simulink model "xmc_sobel_edge_detection"  (R2023a)
settings: Solver=VariableStepAuto  StartTime=0.0  StopTime=inf  RelTol=1e-3  EnableMultiTasking=on
PostLoadFcn:
  | xmcHubUpdateInstalledDevice(gcs);
undefined symbols (not defined in the file): A, AXI4, N, Stream, xc7vx485tffg1157
libraries: visionsinks x3, hlsBasic x3, vmcUtilities x2, sobel_edge_detection_lib x2, dspvision x1, hlsUtilities x1
settings Model: Creator=dvancamp  LastModifiedBy=robg
settings SolverCC: AlgebraicLoopSolver=TrustRegion
settings DataIOCC: LimitDataPoints=on  ReturnWorkspaceOutputs=off
settings OptimizationCC: LifeSpan=inf
settings DebuggingCC: UnconnectedInputMsg=warning  UnconnectedOutputMsg=warning  UnconnectedLineMsg=warning  AllowSymbolicDim=off  SFUnexpectedBacktrackingDiag=warning  SFNoUnconditionalDefaultTransitionDiag=warning  ArithmeticOperatorsInVariantConditions=warning
settings ModelReferenceCC: EnableRefExpFcnMdlSchedulingChecks=on  PropagateSignalLabelsOutOfModel=off
settings SFSimCC: SimUseLocalCustomCode=off  CustomCodeUndefinedFunction=UseInterfaceOnly
settings RTWCC: RTWUseLocalCustomCode=off  DLArmComputeVersion=19.05
settings CodeAppCC: StateflowObjectComments=on
settings GRTTargetCC: TargetLangStandard=C89/C90 (ANSI)
settings ConfigComp: CovMetricSettings=dw  CovSaveCumulativeToWorkspaceVar=on  CovSaveSingleToWorkspaceVar=on  CovExternalEMLEnable=off

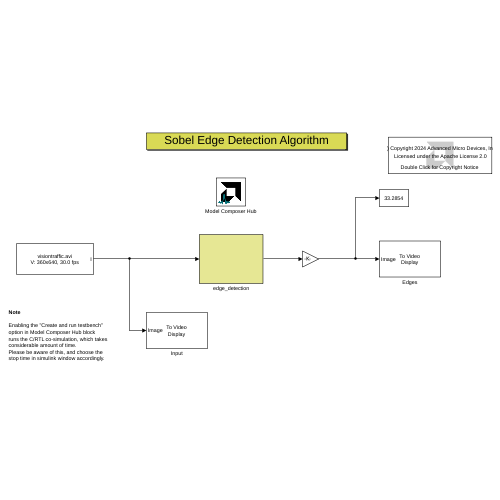
[thumbnail: Simulink's stored preview of the top-level diagram]
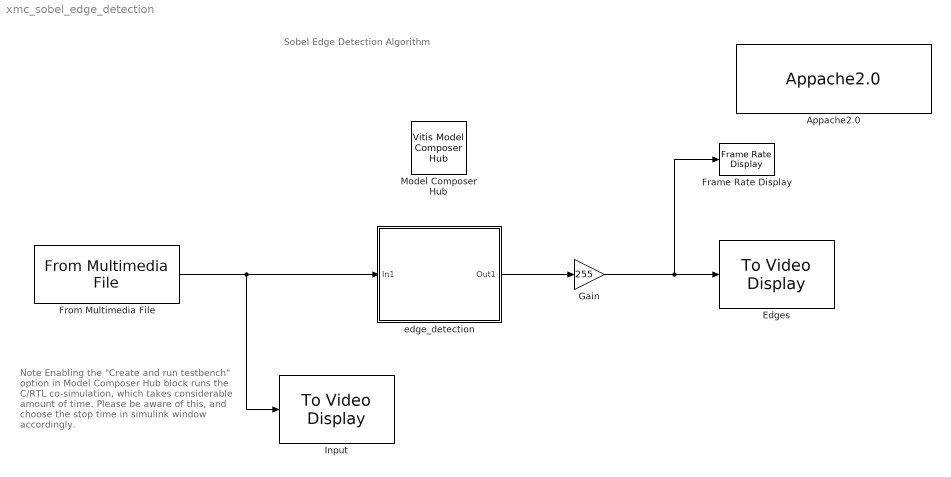
== system xmc_sobel_edge_detection ==
  note: Sobel Edge Detection Algorithm
  note: Note
      |
      | Enabling the "Create and run testbench" option in Model Composer Hub block
      | runs the C/RTL co-simulation, which takes considerable amount of time.
      | Please be aware of this, and choose the stop time in simulink window accordingly.
  Appache2.0 : vmcUtilities/Appache2.0
  Edges : visionsinks/To Video Display  windowSizeMode=True size (1:1)  openAtMdlStart=on  fullScreen=off  videoWindowX=1115  videoWindowY=603  saveWindowSize=off  videoWindowWidth=640  videoWindowHeight=360  inputColorFormat=RGB  inputType=Obsolete  imagePorts=One multidimensional signal  OutputDevice=On-screen video monitor  dataOrg=Column-major  isWindowOpen=off
  Frame Rate Display : visionsinks/Frame Rate Display  UpdateRate=10
  From Multimedia File : dspvision/From Multimedia File  inputFilename=visiontraffic.avi  readRange=[1 Inf]  loop=on  numPlays=inf  outputStreams=Video only  videoDataType=uint8  audioDataType=int16  inheritSampleTime=off  userDefinedSampleTime=1/30  noAudioOutput=off  isIntensityVideo=off  fourcc=Intensity  colorVideoFormat=One multidimensional signal  outputEOF=off  dataOrg=Column-major  audioFrameSize=1024  computeAudioFrameSize=off  outSamplingMode=Sample based
  Gain : Gain  Gain=255  OutDataTypeStr=uint8
  Input : visionsinks/To Video Display  windowSizeMode=Normal  openAtMdlStart=on  fullScreen=off  videoWindowX=194  videoWindowY=606  saveWindowSize=off  videoWindowWidth=613  videoWindowHeight=348  inputColorFormat=RGB  inputType=Obsolete  imagePorts=One multidimensional signal  OutputDevice=On-screen video monitor  dataOrg=Column-major  isWindowOpen=off
  Model Composer Hub : vmcUtilities/Vitis Model Composer Hub  Tag=genX  CodeGeneration=off  SubsystemName=edge_detection  StartColumn=1  NumberOfColumns=1  TargetDirectory=./code  exportDesign=off  analyzeDesign=off  validateDesignOnHw=off  ExportType=IP Catalog  IpVendor=xilinx.com  IpLibrary=hls  IpVersion=1.0  IpHWLanguage=Verilog  AieCompilerOptions={}  AieSimulatorOptions={}  CreateTestbench=off  TestbenchStackSize=10  RunRtlSim=off  RunCSim=off  RunAieSim=off  AieSimTimeout=50000  RunAieSimProfiling=off  LaunchVitisAnalyzer=off  PlotOutput=off  RunX86Sim=on  X86SimTimeout=10  GenHwImage=off  GenLibadfXo=off  GenHwValidationCode=off  PlatformType=Not Specified  HwSystemType=Baremetal  HwValidationTarget=hw  ProjDevice=xc7vx485tffg1157-1  ProjDevicePart=xc7vx485tffg1157-1  SamplePeriod=-1  ClockFrequency=200  DataPathParallelism=1  xilinxfamily=Kintex7  part=xc7k325t  speed=-3  package=fbg676  directory=./netlist  testbench=off  incr_netlist=off  synthesis_tool=Vivado  clock_wrapper=Clock Enables  dbl_ovrd=According to Block Masks  dcm_input_clock_period=10  sysclk_period=10  simulink_period=1  eval_field=0  LogFileName=''  NThreads=4
  edge_detection : Subsystem
  wires:
  edge_detection/1(Out1) -> Gain/1
  Gain/1 -> Edges/1, Frame Rate Display/1
  From Multimedia File/1 -> Input/1, edge_detection/1(In1)

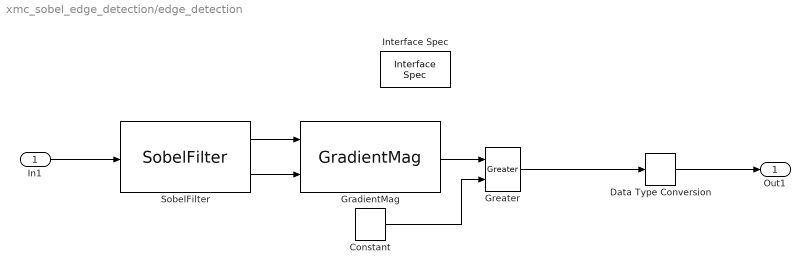
== system xmc_sobel_edge_detection/edge_detection ==
  In1 : Inport
  Constant : hlsBasic/Constant  Value=130  VectorParams1D=off  SampleTime=-1  OutDataType=double  TypeExp=''  Signedness=Signed  WordLength=16  FractionalLength=0  RoundingMode=Truncation to minus infinity  OverflowMode=Wrap around
  Data Type Conversion : hlsBasic/Data Type Conversion  OutDataType=uint8  TypeExp=''  Signedness=Signed  WordLength=16  FractionalLength=0  RoundingMode=Truncation to minus infinity  OverflowMode=Wrap around
  GradientMag : sobel_edge_detection_lib/GradientMag  LibraryFunction=GradientMag  IncludeFiles={'gradient_magnitude_wrap.h'}  SourceFiles={}  IncludeDirectories={'./include'}  TemplateParams={'int ROWS'; 'int COLS'; 'int NPC=1'}  FunctionParamTypes={xmcDataType('void'); xmcDataType('uint16_t'); xmcDataType('uint16_t'); xmcDataType('uint16_t'); xmcDataType('int')}  FunctionParamPassbys={0.000000000000000000e+00; 0.000000000000000000e+00; 0.000000000000000000e+00; 0.000000000000000000e+00; 0.000000000000000000e+00}  FunctionParamDimensions={'1'; '[ROWS][COLS]'; '[ROWS][COLS]'; '[ROWS][COLS]'; '1'}  FunctionParamNames={'return'; 'inX'; 'inY'; 'Out'; 'NPC'}  FunctionParamDir={0.000000000000000000e+00; 1.000000000000000000e+00; 1.000000000000000000e+00; 2.000000000000000000e+00; 3.000000000000000000e+00}  FunctionParamSupportsStreaming={true; true; true; true; true}  BufferDepth={'0'}  FunctionParamValues={'0'; '0'; '0'; '0'; '1'}  ThroughputFactors={''}  NPC=1
  Greater : hlsBasic/Greater
  Interface Spec : hlsUtilities/Interface Spec  Return=AXI4-Lite Slave@@  InportInterfaces={'AXI4-Stream@@@N/A@N/A'}  InportHandles={4.692015136718750000e+03}  InportNames={'In1'}  OutportInterfaces={'AXI4-Stream@@@N/A@N/A'}  OutportHandles={4.712013305664062500e+03}  OutportNames={'Out1'}  Mode=AXI4-Lite Slave  InName1=In1  InMode1=AXI4-Stream  InVFormat1=N/A  InVComponent1=N/A  InMode2=Default  InVFormat2=N/A  InVComponent2=N/A  InMode3=Default  InVFormat3=N/A  InVComponent3=N/A  InMode4=Default  InVFormat4=N/A  InVComponent4=N/A  InMode5=Default  InVFormat5=N/A  InVComponent5=N/A  InMode6=Default  InVFormat6=N/A  InVComponent6=N/A  InMode7=Default  InVFormat7=N/A  InVComponent7=N/A  InMode8=Default  InVFormat8=N/A  InVComponent8=N/A  OutName1=Out1  OutMode1=AXI4-Stream  OutVFormat1=N/A  OutVComponent1=N/A  OutMode2=Default  OutVFormat2=N/A  OutVComponent2=N/A  OutMode3=Default  OutVFormat3=N/A  OutVComponent3=N/A  OutMode4=Default  OutVFormat4=N/A  OutVComponent4=N/A  OutMode5=Default  OutVFormat5=N/A  OutVComponent5=N/A  OutMode6=Default  OutVFormat6=N/A  OutVComponent6=N/A  OutMode7=Default  OutVFormat7=N/A  OutVComponent7=N/A  OutMode8=Default  OutVFormat8=N/A  OutVComponent8=N/A
  SobelFilter : sobel_edge_detection_lib/SobelFilter  LibraryFunction=SobelFilter  IncludeFiles={'sobel_filter_wrap.h'}  SourceFiles={}  IncludeDirectories={'./include'}  TemplateParams={'int ROWS'; 'int COLS'; 'int NPC=1'}  FunctionParamTypes={xmcDataType('void'); xmcDataType('uint8_t'); xmcDataType('uint16_t'); xmcDataType('uint16_t'); xmcDataType('int')}  FunctionParamPassbys={0.000000000000000000e+00; 0.000000000000000000e+00; 0.000000000000000000e+00; 0.000000000000000000e+00; 0.000000000000000000e+00}  FunctionParamDimensions={'1'; '[ROWS][COLS]'; '[ROWS][COLS]'; '[ROWS][COLS]'; '1'}  FunctionParamNames={'return'; 'in'; 'outX'; 'outY'; 'NPC'}  FunctionParamDir={0.000000000000000000e+00; 1.000000000000000000e+00; 2.000000000000000000e+00; 2.000000000000000000e+00; 3.000000000000000000e+00}  FunctionParamSupportsStreaming={true; true; true; true; true}  BufferDepth={'0'}  FunctionParamValues={'0'; '0'; '0'; '0'; '1'}  ThroughputFactors={''}  NPC=1
  Out1 : Outport
  wires:
  In1/1 -> SobelFilter/1
  GradientMag/1 -> Greater/1
  Greater/1 -> Data Type Conversion/1
  Constant/1 -> Greater/2
  SobelFilter/1 -> GradientMag/1
  SobelFilter/2 -> GradientMag/2
  Data Type Conversion/1 -> Out1/1
